simulink model "FOPD_linear_model"  (R2018b)
settings: Solver=ode4  StartTime=0.0  StopTime=10.0  FixedStep=0.01  MaxStep=0.2  RelTol=1e-3
settings Model: Creator=standard  LastModifiedBy=standard

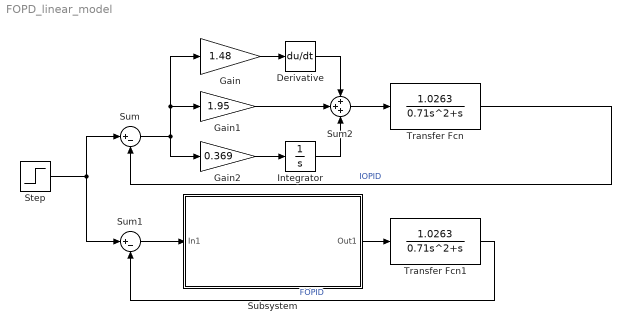
== system FOPD_linear_model ==
  Derivative : Derivative
  Gain : Gain  Gain=1.48
  Gain1 : Gain  Gain=1.95
  Gain2 : Gain  Gain=0.369
  Integrator : Integrator
  Step : Step  SampleTime=0
  Subsystem : Subsystem
  Sum : Sum  Inputs=|+-
  Sum1 : Sum  Inputs=|+-
  Sum2 : Sum  Inputs=+++
  Transfer Fcn : TransferFcn  Numerator=[1.0263]  Denominator=[0.71 1 0]
  Transfer Fcn1 : TransferFcn  Numerator=[1.0263]  Denominator=[0.71 1 0]
  wires:
  Transfer Fcn/1 -> Sum/2  "IOPID"
  Step/1 -> Sum1/1, Sum/1
  Transfer Fcn1/1 -> Sum1/2  "FOPID"
  Sum1/1 -> Subsystem/1(In1)
  Subsystem/1(Out1) -> Transfer Fcn1/1
  Gain/1 -> Derivative/1
  Gain2/1 -> Integrator/1
  Derivative/1 -> Sum2/1
  Integrator/1 -> Sum2/3
  Gain1/1 -> Sum2/2
  Sum/1 -> Gain1/1, Gain/1, Gain2/1
  Sum2/1 -> Transfer Fcn/1

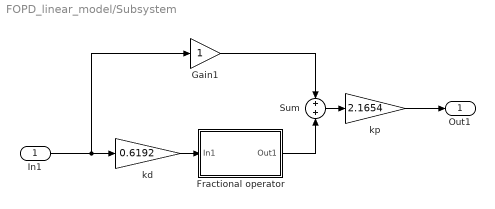
== system FOPD_linear_model/Subsystem ==
  In1 : Inport
  "Fractional operator " : Subsystem  mask{gam=1.0497, ww=[1e-3, 1e3], n=5, kF1=on, kF=Modified Oustaloup filter}
      mask prompts: gam "Derivative order gamma"; ww "Frequency range [wb,wh]"; n "Apprixmation order"; kF1 "Is a low-pass filter required?"; kF "Filter type"
      mask init:
      | wb=ww(1); wh=ww(2); 
      | if kF==1, G=ousta_fod(gam,n,wb,wh);
      | else, G=new_fod(gam,n,wb,wh); end
      | num=G.num{1}; den=G.den{1}; T=1/wh; str='Fractional\n';
      | if isnumeric(gam)
      | 	if gam>0, str=[str, 'Der  s^' num2str(gam) ];
      | 	else, str=[str, 'Int  s^{' num2str(gam) '}']; end
      | else, str=[str, 'Der  s^gam']; end
      | if kF1==1, G=G*tf(1,[T 1]); end
      mask TypeOptions kF: Oustaloup filter | Modified Oustaloup filter | Matsuda-Fujii filter
      mask Display: disp(str)
  Gain1 : Gain
  Sum : Sum
  kd : Gain  Gain=0.6192
  kp : Gain  Gain=2.1654
  Out1 : Outport
  wires:
  In1/1 -> Gain1/1, kd/1
  kd/1 -> "Fractional operator "/1(In1)
  Sum/1 -> kp/1
  "Fractional operator "/1(Out1) -> Sum/2
  Gain1/1 -> Sum/1
  kp/1 -> Out1/1

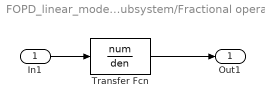
== system FOPD_linear_model/Subsystem/Fractional operator  ==
  In1 : Inport
  Transfer Fcn : TransferFcn  Numerator=num  Denominator=den
  Out1 : Outport
  wires:
  In1/1 -> Transfer Fcn/1
  Transfer Fcn/1 -> Out1/1
